simulink model "StopWatchProject"  (R2016b)
settings: Solver=FixedStepAuto  StartTime=0.0  StopTime=Inf  FixedStep=Auto  RelTol=1e-3  EnableMultiTasking=on
libraries: simulink x1
settings Model: Creator=admim  LastModifiedBy=silviobacci
settings DataIOCC: LimitDataPoints=on  SaveFormat=Array
settings OptimizationCC: DefaultParameterBehavior=Inlined  InlineInvariantSignals=on
settings DebuggingCC: SolverPrmCheckMsg=warning  ParameterTunabilityLossMsg=error  SFUnexpectedBacktrackingDiag=warning  SFNoUnconditionalDefaultTransitionDiag=warning  SFExecutionAtInitializationDiag=none
settings HardwareCC: ProdBitPerPointer=32  ProdBitPerSizeT=32  ProdBitPerPtrDiffT=32  ProdLargestAtomicFloat=None  ProdIntDivRoundTo=Undefined  ProdEndianess=Unspecified  ProdWordSize=32  ProdHWDeviceType=32-bit Generic
settings ModelReferenceCC: PropagateSignalLabelsOutOfModel=off
settings RTWCC: SystemTargetFile=ert.tlc  GenCodeOnly=on  TemplateMakefile=ert_default_tmf  Description=Embedded Coder
settings CodeAppCC: ForceParamTrailComments=on  IgnoreCustomStorageClasses=off  OperatorAnnotations=on  SimulinkDataObjDesc=on  SFDataObjDesc=on  MATLABFcnDesc=on  InsertBlockDesc=on  MATLABSourceComments=on
settings ERTTargetCC: SupportAbsoluteTime=off  MultiInstanceERTCode=on  CodeInterfacePackaging=Reusable function  SupportNonFinite=off  SupportComplex=off  PurelyIntegerCode=on  InlinedParameterPlacement=NonHierarchical  MultiInstanceErrorCode=None  ERTCustomFileTemplate=example_file_process.tlc
settings ConfigComp: CovMetricSettings=dw  CovHtmlReporting=on  CovSaveCumulativeToWorkspaceVar=on  CovSaveSingleToWorkspaceVar=on  CovExternalEMLEnable=off  CovSFcnEnable=off

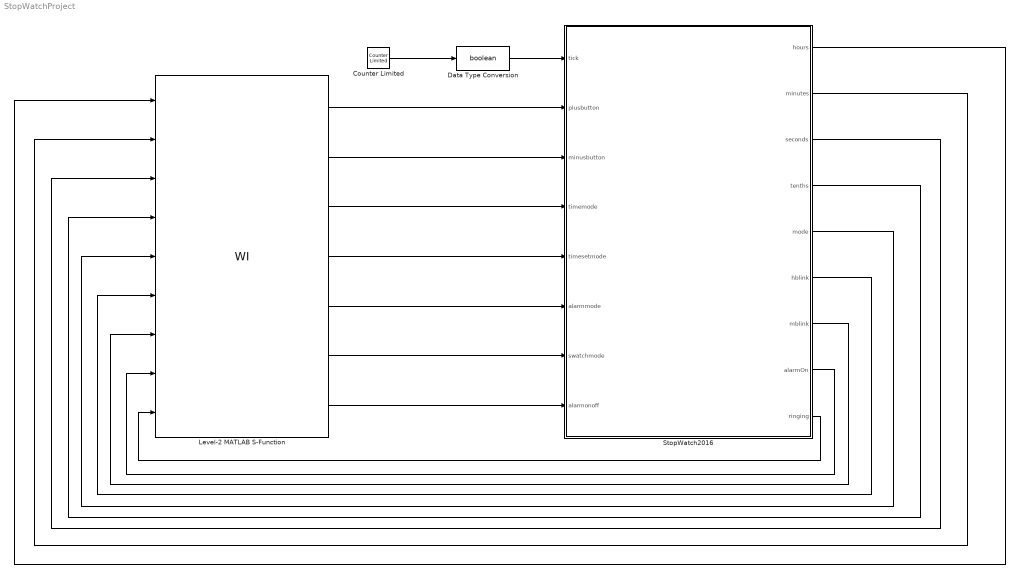
== system StopWatchProject ==
  Counter Limited : simulink/Sources/Counter Limited  uplimit=1  tsamp=60
  Data Type Conversion : DataTypeConversion  OutDataTypeStr=boolean
  Level-2 MATLAB S-Function : M-S-Function  FunctionName=WI
  StopWatch2016 : Subsystem
  wires:
  Counter Limited/1 -> Data Type Conversion/1
  Level-2 MATLAB S-Function/1 -> StopWatch2016/2(plusbutton)
  Level-2 MATLAB S-Function/2 -> StopWatch2016/3(minusbutton)
  Level-2 MATLAB S-Function/3 -> StopWatch2016/4(timemode)
  Level-2 MATLAB S-Function/4 -> StopWatch2016/5(timesetmode)
  Level-2 MATLAB S-Function/5 -> StopWatch2016/6(alarmmode)
  Level-2 MATLAB S-Function/6 -> StopWatch2016/7(swatchmode)
  StopWatch2016/1(hours) -> Level-2 MATLAB S-Function/1
  StopWatch2016/2(minutes) -> Level-2 MATLAB S-Function/2
  StopWatch2016/3(seconds) -> Level-2 MATLAB S-Function/3
  StopWatch2016/4(tenths) -> Level-2 MATLAB S-Function/4
  StopWatch2016/5(mode) -> Level-2 MATLAB S-Function/5
  Level-2 MATLAB S-Function/7 -> StopWatch2016/8(alarmonoff)
  StopWatch2016/6(hblink) -> Level-2 MATLAB S-Function/6
  StopWatch2016/9(ringing) -> Level-2 MATLAB S-Function/9
  StopWatch2016/8(alarmOn) -> Level-2 MATLAB S-Function/8
  StopWatch2016/7(mblink) -> Level-2 MATLAB S-Function/7
  Data Type Conversion/1 -> StopWatch2016/1(tick)

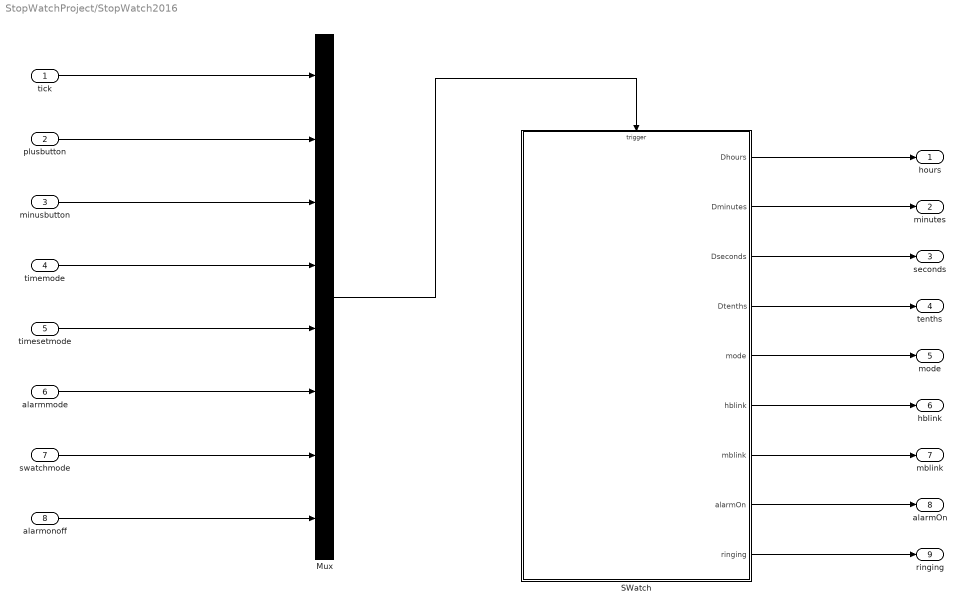
== system StopWatchProject/StopWatch2016 ==
  tick : Inport
  plusbutton : Inport  Port=2
  minusbutton : Inport  Port=3
  timemode : Inport  Port=4
  timesetmode : Inport  Port=5
  alarmmode : Inport  Port=6
  swatchmode : Inport  Port=7
  alarmonoff : Inport  Port=8  OutDataTypeStr=boolean
  Mux : Mux  Inputs=8
  SWatch : Stateflow chart  TreatAsAtomicUnit=on
  hours : Outport
  minutes : Outport  Port=2
  seconds : Outport  Port=3
  tenths : Outport  Port=4
  mode : Outport  Port=5
  hblink : Outport  Port=6  OutDataTypeStr=boolean
  mblink : Outport  Port=7  OutDataTypeStr=boolean
  alarmOn : Outport  Port=8  OutDataTypeStr=boolean
  ringing : Outport  Port=9  OutDataTypeStr=boolean
  wires:
  timesetmode/1 -> Mux/5
  alarmmode/1 -> Mux/6
  timemode/1 -> Mux/4
  minusbutton/1 -> Mux/3
  Mux/1 -> SWatch/Trigger
  SWatch/1(Dhours) -> hours/1
  SWatch/4(Dtenths) -> tenths/1
  SWatch/3(Dseconds) -> seconds/1
  SWatch/2(Dminutes) -> minutes/1
  plusbutton/1 -> Mux/2
  swatchmode/1 -> Mux/7
  SWatch/5(mode) -> mode/1
  SWatch/6(hblink) -> hblink/1
  SWatch/7(mblink) -> mblink/1
  SWatch/8(alarmOn) -> alarmOn/1
  alarmonoff/1 -> Mux/8
  SWatch/9(ringing) -> ringing/1
  tick/1 -> Mux/1

== stateflow chart StopWatchProject/StopWatch2016/SWatch ==
  settings: executeAtInitialization=1
  state Control [parallel]
    settings: executionOrder=1
    state timemode
      en:mode=uint8(0)
      timemode -> timemode [order 1] : ttick{Dhours=hours;Dminutes=minutes;Dseconds=seconds}
    state timesetmode
      entry:mode=uint8(1)
      state sethours
        en:Dhours=hours; Dminutes=minutes; hblink= true;
        ex: hblink= false;
      state setminutes
        en:Dminutes=minutes; mblink= true;
        ex: mblink= false;
      Control.timesetmode.sethours -> Control.timesetmode.sethours [order 3] : Bminus/{hours = hours - 1}
      Control.timesetmode.sethours -> Control.timesetmode.sethours [order 2] : Bminus[hours==0]/{hours= uint8(23)}
      Control.timesetmode.setminutes -> Control.timesetmode.setminutes [order 3] : Bminus/{minutes = minutes - 1}
      Control.timesetmode.setminutes -> Control.timesetmode.setminutes [order 2] : Bminus[minutes==0]/{minutes= uint8(59)}
      Control.timesetmode.sethours -> Control.timesetmode.setminutes [order 4] : Btimeset
      (default) -> Control.timesetmode.sethours
      Control.timesetmode.setminutes -> Control.timesetmode.sethours [order 4] : Btimeset
      Control.timesetmode.sethours -> Control.timesetmode.sethours [order 1] : Bplus/{hours=mod(hours+1,24)}
      Control.timesetmode.setminutes -> Control.timesetmode.setminutes [order 1] : Bplus/{minutes=mod(minutes+1,60)}
    state swatchmode
      en:mode=uint8(3)
      state stopped
        en:Dhours=SWhours;Dminutes=SWminutes;Dseconds=SWseconds;Dtenths=SWtenths;
      state running
        du: if(lapmode==false) Dhours=SWhours;Dminutes=SWminutes;Dseconds=SWseconds;Dtenths=SWtenths; end
        state counting
        counting -> (junction 89) : ttick{SWtenths = mod(SWtenths + 1,10)}
        (junction 89) -> (junction 91) : [SWtenths==0]{SWseconds=mod(SWseconds+1,60)}
        (junction 91) -> (junction 93) : [SWseconds==0]{SWminutes=mod(SWminutes+1,60)}
        (default) -> counting
        (junction 93) -> (junction 95) : [SWminutes==0]{SWhours=mod(SWhours+1,60)}
        (junction 95) -> counting
      (default) -> (junction 113)
      (junction 113) -> stopped : {SWhours= uint8(0); SWminutes= uint8(0); SWseconds= uint8(0); SWtenths= uint8(0);}
      swatchmode -> (junction 113) [order 1] : Bstop
      stopped -> running : Bplus {lapmode= false;}
      running -> stopped [order 4] : Bplus{lapmode= true;}
      running -> running [order 1] : Bminus[lapmode==false]{lapmode= true}
      running -> running [order 2] : Bminus{lapmode= false}
      running -> running [order 3] : Bplus[lapmode==true]{lapmode= false}
    state alarmmode
      en:mode=uint8(2)
      state sethours
        en:Dhours=Ahours; Dminutes=Aminutes; hblink= true;
        ex: hblink= false;
      state setminutes
        en:Dminutes=Aminutes; mblink= true;
        ex: mblink= false;
      Control.alarmmode.sethours -> Control.alarmmode.sethours [order 2] : Bminus[Ahours==0]/{Ahours= uint8(23)}
      Control.alarmmode.sethours -> Control.alarmmode.sethours [order 3] : Bminus/{Ahours = Ahours - 1}
      Control.alarmmode.setminutes -> Control.alarmmode.setminutes [order 3] : Bminus/{Aminutes = Aminutes - 1}
      Control.alarmmode.setminutes -> Control.alarmmode.setminutes [order 2] : Bminus[Aminutes==0]/{Aminutes= uint8(59)}
      Control.alarmmode.sethours -> Control.alarmmode.setminutes [order 4] : Balarm
      (default) -> Control.alarmmode.sethours
      Control.alarmmode.setminutes -> Control.alarmmode.sethours [order 4] : Balarm
      Control.alarmmode.sethours -> Control.alarmmode.sethours [order 1] : Bplus/{Ahours=mod(Ahours+1,24)}
      Control.alarmmode.setminutes -> Control.alarmmode.setminutes [order 1] : Bplus/{Aminutes=mod(Aminutes+1,60)}
    (default) -> timemode : /{hblink=false, mblink= false}
    timemode -> timesetmode [order 1] : Btimeset
    timesetmode -> alarmmode [order 1] : Balarm
    Control -> timemode : Btime
    timemode -> alarmmode [order 3] : Balarm
    timesetmode -> swatchmode [order 2] : Bstop
    swatchmode -> timesetmode [order 1] : Btimeset
    alarmmode -> timesetmode [order 1] : Btimeset
    timemode -> swatchmode [order 2] : Bstop
    alarmmode -> swatchmode [order 2] : Bstop
    swatchmode -> alarmmode [order 2] : Balarm
    alarmmode -> alarmmode [order 4] : BalarmOnOff{alarmOn=false; ringing=false;}
    alarmmode -> alarmmode [order 3] : BalarmOnOff[alarmOn==false]{alarmOn=true}
  state TimeCount [parallel]
    settings: executionOrder=2
    state timecount
    (default) -> timecount : /{hours=uint8(0);minutes=uint8(0);seconds=uint8(0);tenths=uint8(0)}
    timecount -> (junction 20) : ttick {tenths=mod(tenths+1,10)}
    (junction 20) -> (junction 34) [order 2]
    (junction 20) -> (junction 28) [order 1] : [tenths==0]{seconds=mod(seconds+1, 60)}
    (junction 34) -> timecount
    (junction 28) -> (junction 34) [order 2]
    (junction 31) -> (junction 34) [order 2]
    (junction 28) -> (junction 31) [order 1] : [seconds==0]{minutes=mod(minutes+1, 60)}
    (junction 31) -> (junction 36) [order 1] : [minutes==0]{hours=mod(hours+1,24)}
    (junction 36) -> timecount
  state AlarmMng [parallel]
    en:alarmOn=false; ringing=false;
    settings: executionOrder=3
    state silent
    state ringing
      en: ringing=true;
      ex: ringing=false;
    (default) -> silent : {Ahours= uint8(0);Aminutes= uint8(0);}
    silent -> ringing : [alarmOn==true && hours==Ahours && minutes==Aminutes]
    ringing -> silent : [Ahours~=hours || Aminutes~=minutes || ringing==false]
  data: hours local uint8; minutes local uint8; seconds local uint8; tenths local uint8; Dhours output uint8; Dminutes output uint8; Dseconds output uint8; Dtenths output uint8; mode output uint8; SWhours local uint8; SWminutes local uint8; SWseconds local uint8; SWtenths local uint8; Ahours local uint8; Aminutes local uint8; lapmode local boolean; hblink output boolean; mblink output boolean; alarmOn output boolean; ringing output boolean
  events: ttick input EITHER_EDGE_EVENT; Bplus input RISING_EDGE_EVENT; Bminus input RISING_EDGE_EVENT; Btime input RISING_EDGE_EVENT; Btimeset input RISING_EDGE_EVENT; Balarm input RISING_EDGE_EVENT; Bstop input RISING_EDGE_EVENT; BalarmOnOff input RISING_EDGE_EVENT
